simulink model "Artery"  (R2024b)
settings: Solver=VariableStepAuto  StartTime=0.0  StopTime=10.0  RelTol=1e-3
settings Model: Creator=Apeksha  LastModifiedBy=Apeksha

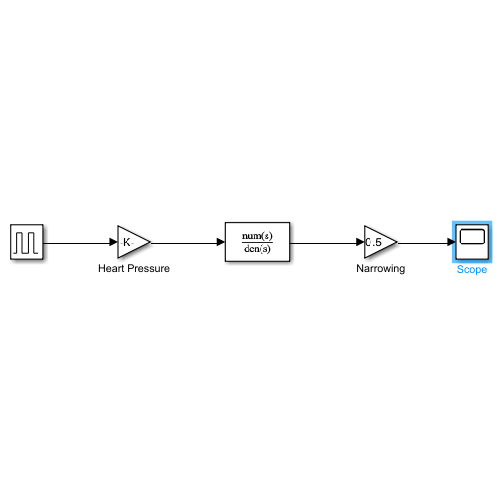
[thumbnail: Simulink's stored preview of the top-level diagram]
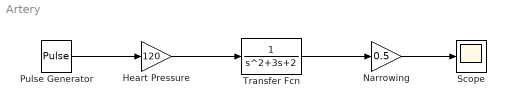
== system Artery ==
  Heart Pressure : Gain  Gain=120
  Narrowing : Gain  Gain=0.5
  Pulse Generator : DiscretePulseGenerator  PulseType=Time based  Period=1  PulseWidth=5
  Scope : Scope
  Transfer Fcn : TransferFcn  Denominator=[1 3 2]
  wires:
  Pulse Generator/1 -> Heart Pressure/1
  Heart Pressure/1 -> Transfer Fcn/1
  Transfer Fcn/1 -> Narrowing/1
  Narrowing/1 -> Scope/1
